simulink model "Traffic_Light"  (R2021a)
settings: Solver=FixedStepDiscrete  StartTime=0.0  StopTime=12  FixedStep=3  RelTol=1e-3  EnableMultiTasking=on
settings Model: Creator=alyma  LastModifiedBy=alyma
settings DataIOCC: ReturnWorkspaceOutputs=off
settings OptimizationCC: DefaultParameterBehavior=Inlined  InlineInvariantSignals=on  EnableMemcpy=off  LifeSpan=1  EfficientTunableParamExpr=on
settings DebuggingCC: UnderspecifiedInitializationDetection=Classic  MergeDetectMultiDrivingBlocksExec=none  SFMachineParentedDataDiag=warning  ArithmeticOperatorsInVariantConditions=warning
settings ModelReferenceCC: PropagateSignalLabelsOutOfModel=off
settings SFSimCC: MATLABDynamicMemAlloc=off  CustomCodeUndefinedFunction=UseInterfaceOnly
settings RTWCC: SystemTargetFile=ert.tlc  GenCodeOnly=on  TemplateMakefile=ert_default_tmf  GenerateReport=on  IncludeHyperlinkInReport=on  LaunchReport=on  GenerateTraceInfo=on  GenerateTraceReport=on  GenerateTraceReportSl=on  GenerateTraceReportSf=on  GenerateTraceReportEml=on
settings CodeAppCC: ForceParamTrailComments=on  IgnoreCustomStorageClasses=off  OperatorAnnotations=on  SimulinkDataObjDesc=on  SFDataObjDesc=on  MATLABFcnDesc=on  InsertBlockDesc=on  StateflowObjectComments=on  MATLABSourceComments=on
settings ERTTargetCC: MultiwordLength=2048  GenerateSampleERTMain=on  InlinedParameterPlacement=NonHierarchical  ERTCustomFileTemplate=example_file_process.tlc

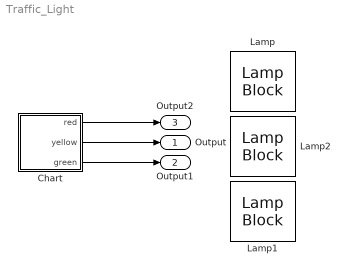
== system Traffic_Light ==
  Chart : Stateflow chart  TreatAsAtomicUnit=on
      settings: PortSchema="{\"entries\":[{\"content\":{\"sides\":[{\"content\":{\"connectorIds\":[]},\"type\":\"ConnectorPlacement.EquallySpacedRectSide\",\"uuid\":\"1467555b-f75e-453d-835a-2323fcd29c80\"},{\"content\":{\"connectorIds\":[\"Out2\",\"Out3\",\"Out1\"],\"side\":\"RIGHT\"},\"type\":\"ConnectorPlacement.EquallySpacedRectSide\",\"uuid\":\"1f1b3075-fb4e-49fa-8547-40d8bc105624\"},{\"content\":{\"connectorIds\":[],\"side\":\"TOP\"},\"type\":\"ConnectorPlacement.EquallySpacedRectSide\",\"uuid\":\"9e7b010d-58c2-4228-a8b3-3fa0eae06258\"}]},\"type\":\"ConnectorPlacement.EquallySpacedConnector\",\"uuid\":\"5ec8d3b2-3c65-4d22-a389-08086ca3b7ff\"}],\"packageUris\":[\"http://schema.mathworks.com/mf0/Connector/R2020b\"],\"version\":\"1.0\"}"
  Lamp : LampBlock
  Lamp1 : LampBlock
  Lamp2 : LampBlock
  Output : Outport
  Output1 : Outport  Port=2
  Output2 : Outport  Port=3  SignalName=RED
  wires:
  Chart/2(red) -> Output2/1
  Chart/1(green) -> Output1/1
  Chart/3(yellow) -> Output/1

== stateflow chart Traffic_Light/Chart ==
  state Stop
    entry:
    red = 1;
    yellow = 0;
    green = 0;
  state PrepareToStop
    entry:
    red = 0;
    yellow = 1;
    green = 0;
  state PrepareToStart
    entry:
    red = 0;
    yellow = 1;
    green = 0;
  state Go
    entry:
    red = 0;
    yellow = 0;
    green = 1;
  (default) -> Stop
  PrepareToStart -> Stop : after(3,sec)
  Stop -> PrepareToStop : after(3,sec)
  PrepareToStop -> Go : after(3,sec)
  Go -> PrepareToStart : after(3,sec)
  data: green output; red output; yellow output
